simulink model "MARCH_v1_4"  (R2016a)
settings: Solver=FixedStepDiscrete  StartTime=0.0  StopTime=inf  FixedStep=0.001  RelTol=1e-3
PostLoadFcn:
  | build_location = fullfile(fileparts(which(bdroot)),'build');
  | 
  | set_param(0, 'CacheFolder', build_location);
  | set_param(0, 'CodeGenFolder', build_location);
InitFcn:
  | % Change dir to model location
  | cd(fileparts(which(bdroot)));
  | 
  | % Run init script
  | init_model;
  | 
  | load db.mat
  | initialize_model_param
StartFcn:
  | % Make sure we always move back to model folder
  | cd(fileparts(which(bdroot)));
StopFcn:
  | % Make sure we always move back to model folder
  | cd(fileparts(which(bdroot)));
model workspace (MAT data in the model file):
  localValue = 1
  targetValue = 0
libraries: xpcethercatlib x57, slrtlib x7, dspnetwork x1, aerolibanimutils x1
(part 1 of 2)
CloseFcn:
  | % Make sure we always move back to model folder
  | cd(fileparts(which(bdroot)));
  | 
  | set_param(0, 'CacheFolder', '');
  | set_param(0, 'CodeGenFolder', '');
PauseFcn:
  | % Make sure we always move back to model folder
  | cd(fileparts(which(bdroot)));
ContinueFcn:
  | % Make sure we always move back to model folder
  | cd(fileparts(which(bdroot)));
settings Model: Creator=rtheyyun  LastModifiedBy=rafae
settings SolverCC: EnableConcurrentExecution=on  ConcurrentTasks=on
settings DataIOCC: LimitDataPoints=on  SaveFinalState=on  SaveFormat=StructureWithTime  SignalLoggingSaveFormat=ModelDataLogs  InspectSignalLogs=on
settings OptimizationCC: BlockReduction=off  OptimizeBlockIOStorage=off  BufferReuse=off  GlobalBufferReuse=off  ExpressionFolding=off  ExpressionDepthLimit=2147483647  LocalBlockOutputs=off
settings DebuggingCC: ReadBeforeWriteMsg=DisableAll  WriteAfterWriteMsg=DisableAll  WriteAfterReadMsg=DisableAll  UnderspecifiedInitializationDetection=Classic  MergeDetectMultiDrivingBlocksExec=none  SolverPrmCheckMsg=warning  InheritedTsInSrcMsg=none  FcnCallInpInsideContextMsg=UseLocalSettings  AllowSymbolicDim=off  StateNameClashWarn=warning
settings HardwareCC: ProdBitPerPointer=32  ProdLargestAtomicFloat=None  ProdWordSize=32  ProdLongLongMode=on  ProdHWDeviceType=Generic->32-bit x86 compatible
settings ModelReferenceCC: UpdateModelReferenceTargets=Force  PropagateSignalLabelsOutOfModel=off
settings RTWCC: SystemTargetFile=slrt.tlc  TemplateMakefile=slrt_default_tmf  Description=Simulink Real-Time  RTWVerbose=off
settings TargetCC: CodeReplacementLibrary=XPC_BLAS  ParMdlRefBuildCompliant=on  ConcurrentExecutionCompliant=on  MatFileLogging=on  MATLABClassNameForMDSCustomization=xpcAperiodicCustomization
settings ConfigComp: CovModelRefEnable=Off  CovSFcnEnable=off

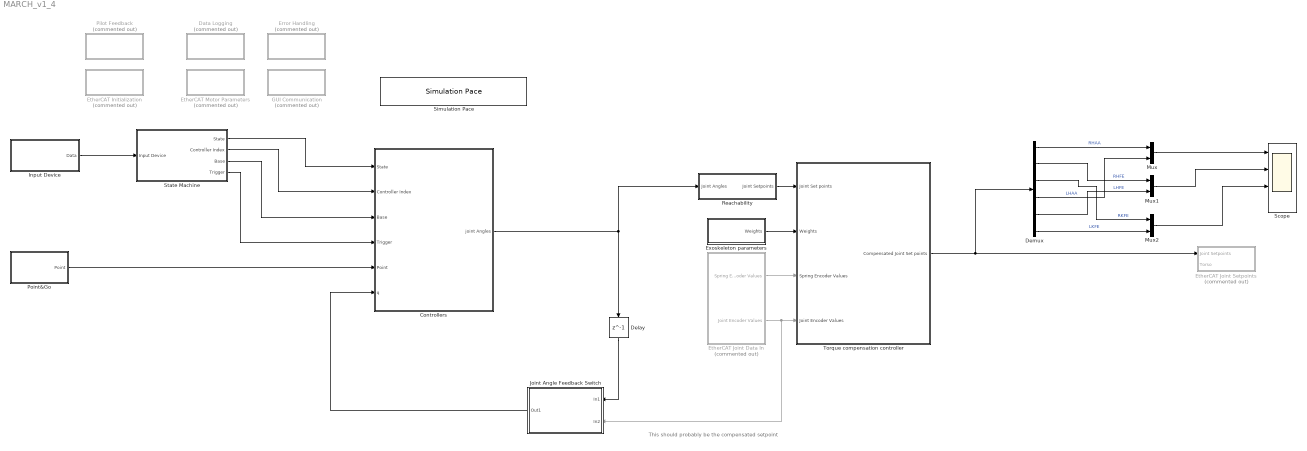
== system MARCH_v1_4 ==
  note: This should probably be the compensated setpoint
  Controllers : Subsystem
  Data Logging : Subsystem  Commented=on
  Delay : Delay  DelayLength=1
  Demux : Demux  Outputs=6
  Error Handling : Subsystem  Commented=on
  EtherCAT Initialization : Subsystem  Commented=on
  EtherCAT Joint Data In : Subsystem  Commented=on
  EtherCAT Joint Setpoints : Subsystem  Commented=on
  EtherCAT Motor Parameters : Subsystem  Commented=on
  Exoskeleton parameters : Subsystem
  GUI Communication : Subsystem  Commented=on
  Input Device : Subsystem
  Joint Angle Feedback Switch : Subsystem
  Mux : Mux  Inputs=2
  Mux1 : Mux  Inputs=2
  Mux2 : Mux  Inputs=2
  Pilot Feedback : Subsystem  Commented=on
  Point&Go : Subsystem
  Reachability : Subsystem
  Scope : Scope  NumInputPorts=4
  Simulation Pace : aerolibanimutils/Simulation Pace  SimulationPace=1  SleepMode=MATLAB Thread  OutputPaceError=off  SampleTime=-1
  State Machine : Subsystem
  Torque compensation controller : Subsystem
  wires:
  Reachability/1(Joint Setpoints) -> Torque compensation controller/1(Joint Set points)
  State Machine/1(State) -> Controllers/1(State)
  EtherCAT Joint Data In/1(Spring Encoder Values) -> Torque compensation controller/3(Spring Encoder Values)
  EtherCAT Joint Data In/2(Joint Encoder Values) -> Joint Angle Feedback Switch/2(In2), Torque compensation controller/4(Joint Encoder Values)
  Exoskeleton parameters/1(Weights) -> Torque compensation controller/2(Weights)
  Controllers/1(joint Angles) -> Reachability/1(Joint Angles), Delay/1
  Joint Angle Feedback Switch/1(Out1) -> Controllers/6(q)
  Delay/1 -> Joint Angle Feedback Switch/1(In1)
  Point&Go/1(Point) -> Controllers/5(Point)
  State Machine/2(Controller Index) -> Controllers/2(Controller Index)
  State Machine/3(Base) -> Controllers/3(Base)
  Input Device/1(Data) -> State Machine/1(Input Device)
  State Machine/4(Trigger) -> Controllers/4(Trigger)
  ? -> Scope/4
  Torque compensation controller/1(Compensated Joint Set points) -> Demux/1, EtherCAT Joint Setpoints/1(Joint Setpoints)
  Demux/1 -> Mux/1  "RHAA"
  Demux/4 -> Mux/2  "LHAA"
  Demux/2 -> Mux1/1  "RHFE"
  Demux/5 -> Mux1/2  "LHFE"
  Demux/3 -> Mux2/1  "RKFE"
  Demux/6 -> Mux2/2  "LKFE"
  Mux/1 -> Scope/1
  Mux1/1 -> Scope/2
  Mux2/1 -> Scope/3

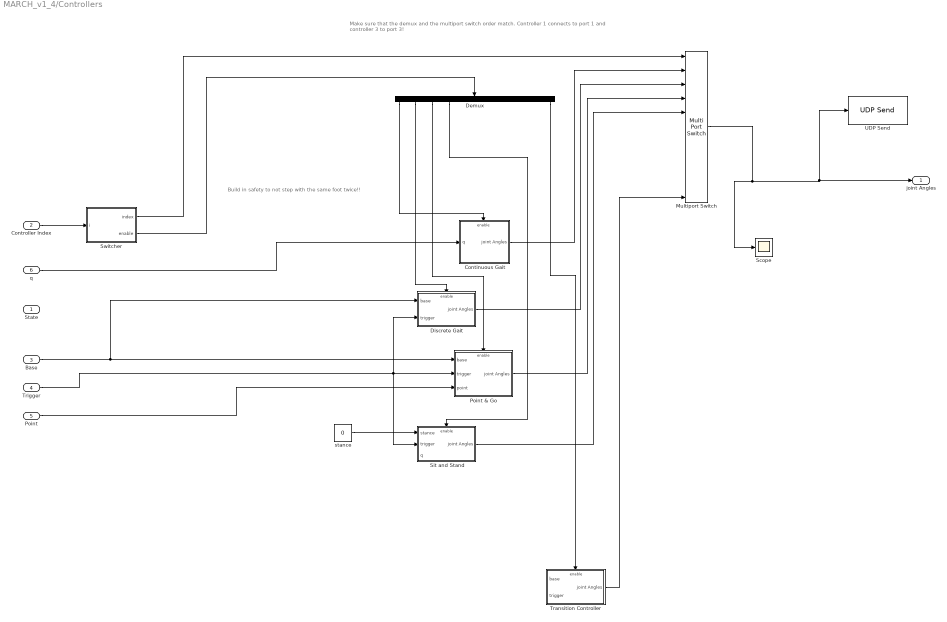
== system MARCH_v1_4/Controllers ==
  note: Build in safety to not step with the same
      | foot twice!!
  note: Make sure that the demux and the multiport switch order match.
      | Controller 1 connects to port 1 and controller 3 to port 3!
  State : Inport
  Controller Index : Inport  Port=2
  Base : Inport  Port=3
  Trigger : Inport  Port=4
  Point : Inport  Port=5
  q : Inport  Port=6
  Continuous Gait : Subsystem
  Demux : Demux  Outputs=10
  Discrete Gait : Subsystem
  Multiport Switch : MultiPortSwitch  Inputs=10
  Point & Go : Subsystem
  Scope : Scope
  Sit and Stand : Subsystem
  Switcher : MATLAB Function  TreatAsAtomicUnit=on
  Transition Controller : Subsystem
  UDP Send : dspnetwork/UDP Send  remoteURL='127.0.0.1'  remotePort=25000  localURL='0.0.0.0'  localPortSource=Automatically determine  localPort=-1  sampletime=-1  separateLengthPort=0
  stance : Constant  Value=0
  joint Angles : Outport
  wires:
  q/1 -> Continuous Gait/1(q)
  Demux/1 -> Continuous Gait/Enable
  Demux/2 -> Discrete Gait/Enable
  Discrete Gait/1(joint Angles) -> Multiport Switch/3
  Controller Index/1 -> Switcher/1(i)
  Switcher/1(index) -> Multiport Switch/1
  Continuous Gait/1(joint Angles) -> Multiport Switch/2
  Multiport Switch/1 -> Scope/1, joint Angles/1, UDP Send/1
  Trigger/1 -> Discrete Gait/2(trigger), Sit and Stand/2(trigger), Point & Go/2(trigger)
  Switcher/2(enable) -> Demux/1
  Base/1 -> Discrete Gait/1(base), Point & Go/1(base)
  Transition Controller/1(joint Angles) -> Multiport Switch/11
  Point & Go/1(joint Angles) -> Multiport Switch/4
  Point/1 -> Point & Go/3(point)
  Demux/3 -> Point & Go/Enable
  Demux/10 -> Transition Controller/Enable
  Demux/4 -> Sit and Stand/Enable
  Sit and Stand/1(joint Angles) -> Multiport Switch/5
  stance/1 -> Sit and Stand/1(stance)

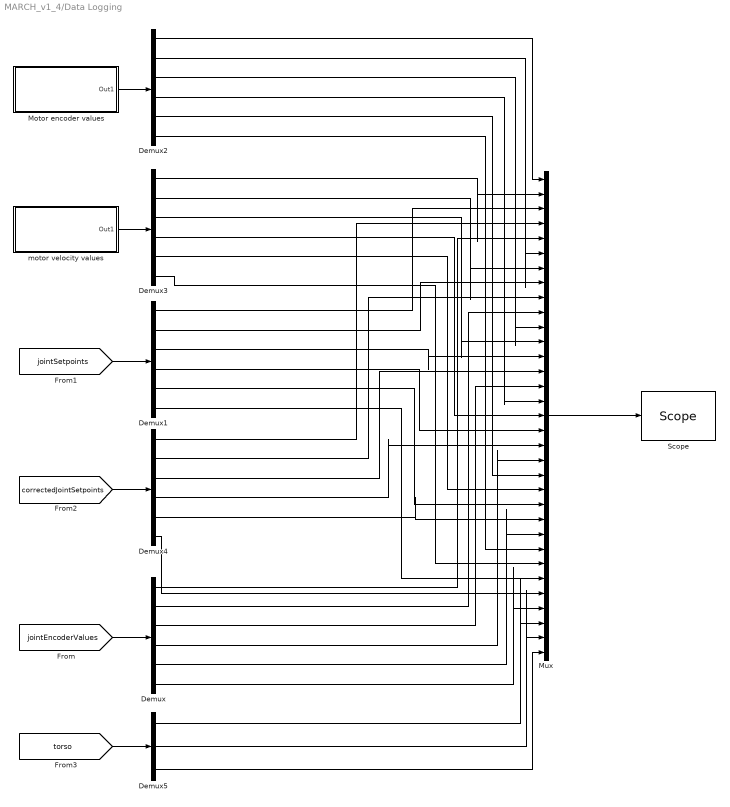
== system MARCH_v1_4/Data Logging ==
  Demux{,1..4} (5 alike) : Demux  Outputs=6
  Demux5 : Demux  Outputs=3
  Motor encoder values : Subsystem
  Mux : Mux  Inputs=33
  "Scope " : slrtlib/Displays and Logging/Scope   scopeno=5  scopetype=File  autostart=on  viewmode=Numerical  formatstr='%15.6f'  grid=on  ylimits=[0,0]  nosamples=250000  noprepostsamples=0  interleave=1  triggermode=FreeRun  triggersignal=1  trigsignalfromport=off  triggerlevel=0.0  triggerslope=Either  triggerscope=1  triggersample=0  filename=datalog.dat  mode=Lazy  writesize=512  autorestart=off  dynamicfilemode=off  maxwritefilesize=512*1024^2
  motor velocity values : Subsystem
  wires:
  Mux/1 -> "Scope "/1
  [jointEncoderValues] -> Demux/1
  [jointSetpoints] -> Demux1/1
  Motor encoder values/1(Out1) -> Demux2/1
  motor velocity values/1(Out1) -> Demux3/1
  Demux2/1 -> Mux/1
  Demux3/1 -> Mux/2
  [correctedJointSetpoints] -> Demux4/1
  [torso] -> Demux5/1
  Demux1/1 -> Mux/3
  Demux4/1 -> Mux/4
  Demux/1 -> Mux/5
  Demux2/2 -> Mux/6
  Demux3/2 -> Mux/7
  Demux1/2 -> Mux/8
  Demux4/2 -> Mux/9
  Demux/2 -> Mux/10
  Demux2/3 -> Mux/11
  Demux3/3 -> Mux/12
  Demux1/3 -> Mux/13
  Demux4/3 -> Mux/14
  Demux/3 -> Mux/15
  Demux2/4 -> Mux/16
  Demux2/6 -> Mux/26
  Demux3/4 -> Mux/17
  Demux1/4 -> Mux/18
  Demux4/4 -> Mux/19
  Demux/4 -> Mux/20
  Demux2/5 -> Mux/21
  Demux3/5 -> Mux/22
  Demux1/5 -> Mux/23
  Demux4/5 -> Mux/24
  Demux/5 -> Mux/25
  Demux3/6 -> Mux/27
  Demux1/6 -> Mux/28
  Demux5/3 -> Mux/33
  Demux5/2 -> Mux/32
  Demux5/1 -> Mux/31
  Demux/6 -> Mux/30
  Demux4/6 -> Mux/29

== system MARCH_v1_4/Error Handling ==

== system MARCH_v1_4/EtherCAT Initialization ==
  "EtherCAT Init " : xpcethercatlib/EtherCAT Init   Priority=0  config_file=D:\Software\MATLAB\simulink-models\EtherCAT Config files\quad_slave_both_legs_v1.0.xml  device_id=0  pci_bus=2  pci_slot=0  dctuning=0  enaDebug=off  enaDC=on  errLink=off  masterDbg=off  stateChgDbg=off  baseClock=off  masterCfg=off  logFile='c:\dbglog.txt'  sample_time=0.001000
  Terminator : Terminator
  wires:
  "EtherCAT Init "/1 -> Terminator/1

== system MARCH_v1_4/EtherCAT Joint Data In ==
  Data Type Conversion : DataTypeConversion  OutDataTypeStr=double
  Joint Encoder EtherCAT : Subsystem  Commented=on
  MATLAB Function : MATLAB Function  TreatAsAtomicUnit=on
  Scope 1 : slrtlib/Displays and Logging/Scope   Commented=on  scopeno=8  scopetype=Target  autostart=on  viewmode=Numerical  formatstr='%15.6f'  grid=on  ylimits=[0,0]  nosamples=3  noprepostsamples=0  interleave=1  triggermode=FreeRun  triggersignal=1  trigsignalfromport=off  triggerlevel=0.0  triggerslope=Either  triggerscope=1  triggersample=0  filename=data.dat  mode=Lazy  writesize=512  autorestart=off  dynamicfilemode=off  maxwritefilesize=512*1024^2
  Scope 2 : slrtlib/Displays and Logging/Scope   Commented=on  scopeno=3  scopetype=Target  autostart=on  viewmode=Numerical  formatstr='%15.6f'  grid=on  ylimits=[0,0]  nosamples=3  noprepostsamples=0  interleave=1  triggermode=FreeRun  triggersignal=1  trigsignalfromport=off  triggerlevel=0.0  triggerslope=Either  triggerscope=1  triggersample=0  filename=data.dat  mode=Lazy  writesize=512  autorestart=off  dynamicfilemode=off  maxwritefilesize=512*1024^2
  Spring Encoder EtherCAT : Subsystem  Commented=on
  Spring Encoder Values : Outport
  Joint Encoder Values : Outport  Port=2
  tag scope: jointEncoderValues=global
  wires:
  Spring Encoder EtherCAT/1(Spring Encoder Values) -> Spring Encoder Values/1
  Joint Encoder EtherCAT/1(Joint Encoder Values) -> Data Type Conversion/1, Scope 2/1, [jointEncoderValues]
  MATLAB Function/1(angles) -> Scope 1/1, Joint Encoder Values/1
  Data Type Conversion/1 -> MATLAB Function/1(encoderValue)

== system MARCH_v1_4/EtherCAT Joint Setpoints ==
  Joint Setpoints : Inport
  Torso : Inport  Port=2
  Subsystem : Subsystem
  exoskeleton : Subsystem
  wires:
  Joint Setpoints/1 -> exoskeleton/1(Joint setpoints), Subsystem/1(Joint Setpoints)
  Torso/1 -> Subsystem/2(Torso)

== system MARCH_v1_4/EtherCAT Motor Parameters ==
  LHFE : Subsystem
  LKFE : Subsystem
  RHFE : Subsystem
  RKFE : Subsystem

== system MARCH_v1_4/Exoskeleton parameters ==
  Constant : Constant
  Weights : Outport
  wires:
  Constant/1 -> Weights/1

== system MARCH_v1_4/GUI Communication ==

== system MARCH_v1_4/Input Device ==
  EtherCAT Input Device : Subsystem  Commented=on
  Left Safety : Constant  Value=0
  Left Trigger : Constant  Value=0
  Local : Constant  Value=localValue
  Mux : Mux  Inputs=6
  Right Safety : Constant  Value=0
  Right Scroll Click : Constant  Value=0
  Right Scroll Position : Constant
  Right Trigger : Constant  Value=0
  Switch : Switch  Criteria=u2 ~= 0
  Data : Outport
  wires:
  Right Scroll Position/1 -> Mux/4
  Mux/1 -> Switch/1
  Right Trigger/1 -> Mux/1
  Switch/1 -> Data/1
  Right Safety/1 -> Mux/2
  Right Scroll Click/1 -> Mux/3
  Left Trigger/1 -> Mux/5
  Local/1 -> Switch/2
  Left Safety/1 -> Mux/6
  EtherCAT Input Device/1(Input Device) -> Switch/3

== system MARCH_v1_4/Joint Angle Feedback Switch ==
  In1 : Inport
  In2 : Inport  Port=2
  Local : Constant  Value=localValue
  Switch : Switch  Criteria=u2 ~= 0
  Out1 : Outport
  wires:
  In2/1 -> Switch/3
  Switch/1 -> Out1/1
  In1/1 -> Switch/1
  Local/1 -> Switch/2

== system MARCH_v1_4/Pilot Feedback ==

== system MARCH_v1_4/Point&Go ==
  EtherCAT Point&Go : Subsystem  Commented=on
  Local : Constant  Value=localValue
  Point & Go Point : Constant  Value=[0.7 -0.3]
  Switch : Switch  Criteria=u2 ~= 0
  Point : Outport
  wires:
  EtherCAT Point&Go/1(Point&Go Data) -> Switch/3
  Local/1 -> Switch/2
  Switch/1 -> Point/1
  Point & Go Point/1 -> Switch/1

== system MARCH_v1_4/Reachability ==
  Joint Angles : Inport
  Data Type Conversion : DataTypeConversion  OutDataTypeStr=uint32
  MATLAB Function : MATLAB Function  Commented=on  TreatAsAtomicUnit=on
  Terminator2 : Terminator
  Joint Setpoints : Outport
  tag scope: jointSetpoints=global
  wires:
  MATLAB Function/2(err) -> Terminator2/1
  Data Type Conversion/1 -> [jointSetpoints]
  Joint Angles/1 -> Data Type Conversion/1, Joint Setpoints/1

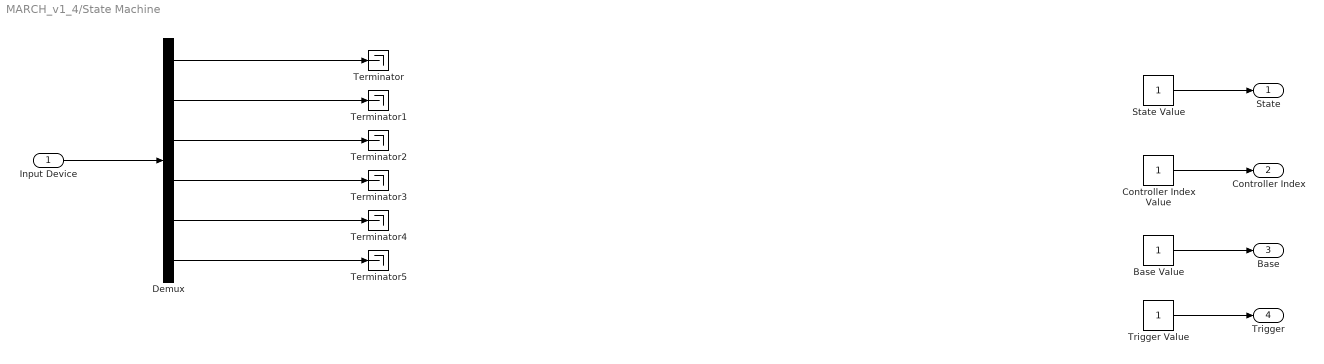
== system MARCH_v1_4/State Machine ==
  Input Device : Inport
  Base Value : Constant
  Controller Index Value : Constant
  Demux : Demux  Outputs=6
  State Value : Constant
  Terminator{,1..5} (6 alike) : Terminator
  Trigger Value : Constant
  State : Outport
  Controller Index : Outport  Port=2
  Base : Outport  Port=3
  Trigger : Outport  Port=4
  wires:
  State Value/1 -> State/1
  Input Device/1 -> Demux/1
  Controller Index Value/1 -> Controller Index/1
  Base Value/1 -> Base/1
  Trigger Value/1 -> Trigger/1
  Demux/1 -> Terminator/1
  Demux/2 -> Terminator1/1
  Demux/3 -> Terminator2/1
  Demux/4 -> Terminator3/1
  Demux/5 -> Terminator4/1
  Demux/6 -> Terminator5/1

== system MARCH_v1_4/Torque compensation controller ==
  Joint Set points : Inport
  Weights : Inport  Port=2
  Spring Encoder Values : Inport  Port=3
  Joint Encoder Values : Inport  Port=4
  Terminator : Terminator
  Terminator1 : Terminator
  Terminator2 : Terminator
  Compensated Joint Set points : Outport
  wires:
  Joint Set points/1 -> Compensated Joint Set points/1
  Joint Encoder Values/1 -> Terminator2/1
  Spring Encoder Values/1 -> Terminator1/1
  Weights/1 -> Terminator/1

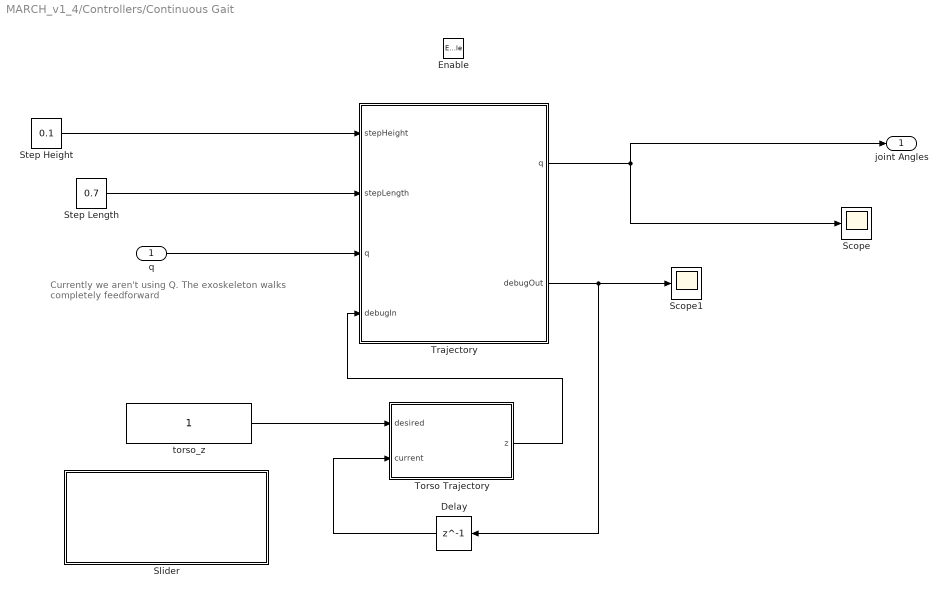
== system MARCH_v1_4/Controllers/Continuous Gait ==
  note: Currently we aren't using Q. The exoskeleton walks completely feedforward
  q : Inport
  Enable : EnablePort
  Delay : Delay  DelayLength=1  InitialCondition=1
  Scope : Scope
  Scope1 : Scope
  Slider : Subsystem  DialogController=hmiCreateDDGDialog  IsWebBlock=on  mask(MWDashboardBlock){webBlockId=08960381-2fc9-439b-949a-5d55ec4678c5, webBlockType=slider, ShowInLibBrowser=on, ShowInitialText=on, HMISrcModelName=MARCH_v1_4}
      mask prompts: webBlockId "WebBlock Id"; webBlockType "WebBlock Type"; HMISrcModelName "Source Model"
      mask Help: helpview([docroot '/mapfiles/simulink.map'], 'hmi_slider')
      mask Display:
      | if strcmp(get_param(bdroot(gcb),'BlockDiagramType'), 'library')
      |     image([(matlabroot) '/toolbox/simulink/hmi/icons/Slider.png']);
      | end
  Step Height : Constant  Value=0.1
  Step Length : Constant  Value=0.7
  Torso Trajectory : MATLAB Function  TreatAsAtomicUnit=on
  Trajectory : MATLAB Function  TreatAsAtomicUnit=on
  torso_z : Constant
  joint Angles : Outport
  wires:
  Step Length/1 -> Trajectory/2(stepLength)
  Trajectory/1(q) -> joint Angles/1, Scope/1
  q/1 -> Trajectory/3("q ")
  Step Height/1 -> Trajectory/1(stepHeight)
  Trajectory/2(debugOut) -> Delay/1, Scope1/1
  torso_z/1 -> Torso Trajectory/1(desired)
  Torso Trajectory/1(z) -> Trajectory/4(debugIn)
  Delay/1 -> Torso Trajectory/2(current)

== system MARCH_v1_4/Controllers/Discrete Gait ==
  base : Inport
  trigger : Inport  Port=2
  Enable : EnablePort
  Delay : Delay  DelayLength=1  InitialCondition=1
  Scope : Scope
  Scope1 : Scope
  Slider : Subsystem  DialogController=hmiCreateDDGDialog  IsWebBlock=on  mask(MWDashboardBlock){webBlockId=bfbe03fb-e7b8-42bf-a623-efab1dfdd155, webBlockType=slider, ShowInLibBrowser=on, ShowInitialText=on, HMISrcModelName=MARCH_v1_4}
      mask prompts: webBlockId "WebBlock Id"; webBlockType "WebBlock Type"; HMISrcModelName "Source Model"
      mask Help: helpview([docroot '/mapfiles/simulink.map'], 'hmi_slider')
      mask Display:
      | if strcmp(get_param(bdroot(gcb),'BlockDiagramType'), 'library')
      |     image([(matlabroot) '/toolbox/simulink/hmi/icons/Slider.png']);
      | end
  Torso Trajectory : MATLAB Function  TreatAsAtomicUnit=on
  Trajectory : MATLAB Function  TreatAsAtomicUnit=on
  torso_z : Constant
  joint Angles : Outport
  wires:
  Trajectory/1(q) -> joint Angles/1, Scope/1
  trigger/1 -> Trajectory/2(trigger)
  Trajectory/2(debugOut) -> Delay/1, Scope1/1
  torso_z/1 -> Torso Trajectory/1(desired)
  Torso Trajectory/1(z) -> Trajectory/4(debugIn)
  Delay/1 -> Torso Trajectory/2(current)
  base/1 -> Trajectory/1(base)

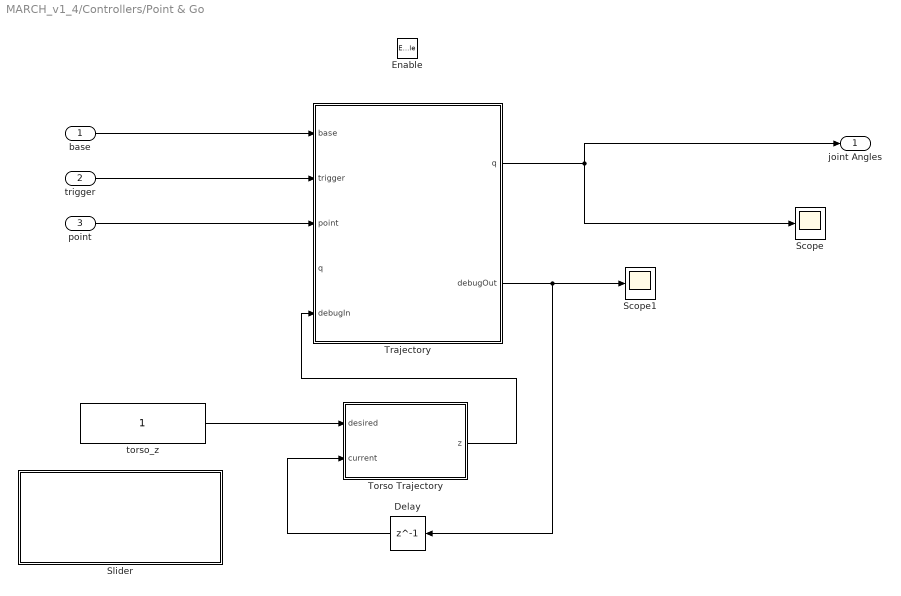
== system MARCH_v1_4/Controllers/Point & Go ==
  base : Inport
  trigger : Inport  Port=2
  point : Inport  Port=3
  Enable : EnablePort
  Delay : Delay  DelayLength=1  InitialCondition=1
  Scope : Scope
  Scope1 : Scope
  Slider : Subsystem  DialogController=hmiCreateDDGDialog  IsWebBlock=on  mask(MWDashboardBlock){webBlockId=86d33f0a-5aea-492b-afd2-e04e6c4ab60f, webBlockType=slider, ShowInLibBrowser=on, ShowInitialText=on, HMISrcModelName=MARCH_v1_4}
      mask prompts: webBlockId "WebBlock Id"; webBlockType "WebBlock Type"; HMISrcModelName "Source Model"
      mask Help: helpview([docroot '/mapfiles/simulink.map'], 'hmi_slider')
      mask Display:
      | if strcmp(get_param(bdroot(gcb),'BlockDiagramType'), 'library')
      |     image([(matlabroot) '/toolbox/simulink/hmi/icons/Slider.png']);
      | end
  Torso Trajectory : MATLAB Function  TreatAsAtomicUnit=on
  Trajectory : MATLAB Function  TreatAsAtomicUnit=on
  torso_z : Constant
  joint Angles : Outport
  wires:
  Trajectory/1(q) -> joint Angles/1, Scope/1
  trigger/1 -> Trajectory/2(trigger)
  Trajectory/2(debugOut) -> Delay/1, Scope1/1
  torso_z/1 -> Torso Trajectory/1(desired)
  Torso Trajectory/1(z) -> Trajectory/5(debugIn)
  Delay/1 -> Torso Trajectory/2(current)
  base/1 -> Trajectory/1(base)
  point/1 -> Trajectory/3(point)

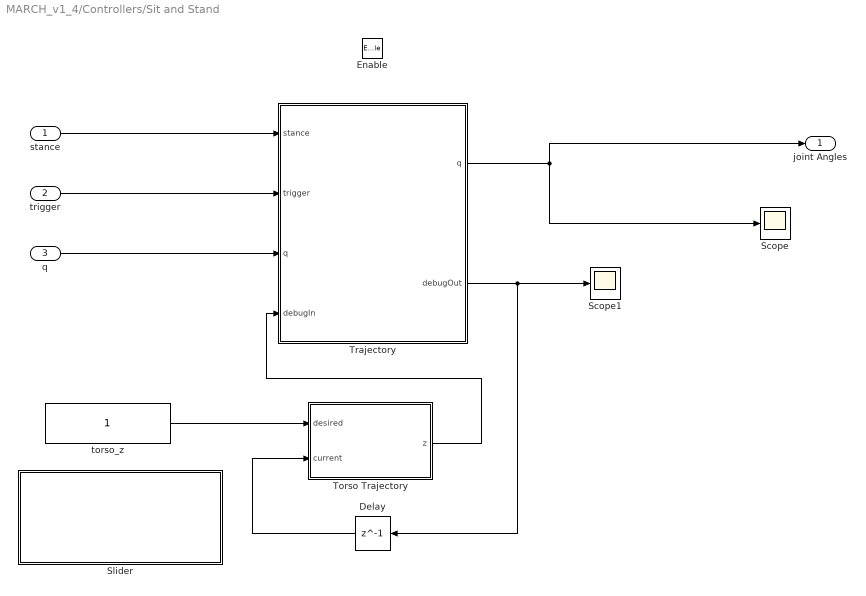
== system MARCH_v1_4/Controllers/Sit and Stand ==
  stance : Inport
  trigger : Inport  Port=2
  "q " : Inport  Port=3
  Enable : EnablePort
  Delay : Delay  DelayLength=1  InitialCondition=1
  Scope : Scope
  Scope1 : Scope
  Slider : Subsystem  DialogController=hmiCreateDDGDialog  IsWebBlock=on  mask(MWDashboardBlock){webBlockId=b1d2559e-7f74-4a22-bcb5-6ee8e71e9ba8, webBlockType=slider, ShowInLibBrowser=on, ShowInitialText=on, HMISrcModelName=MARCH_v1_4}
      mask prompts: webBlockId "WebBlock Id"; webBlockType "WebBlock Type"; HMISrcModelName "Source Model"
      mask Help: helpview([docroot '/mapfiles/simulink.map'], 'hmi_slider')
      mask Display:
      | if strcmp(get_param(bdroot(gcb),'BlockDiagramType'), 'library')
      |     image([(matlabroot) '/toolbox/simulink/hmi/icons/Slider.png']);
      | end
  Torso Trajectory : MATLAB Function  TreatAsAtomicUnit=on
  Trajectory : MATLAB Function  TreatAsAtomicUnit=on
  torso_z : Constant
  joint Angles : Outport
  wires:
  Trajectory/1(q) -> joint Angles/1, Scope/1
  trigger/1 -> Trajectory/2(trigger)
  Trajectory/2(debugOut) -> Delay/1, Scope1/1
  torso_z/1 -> Torso Trajectory/1(desired)
  Torso Trajectory/1(z) -> Trajectory/4(debugIn)
  Delay/1 -> Torso Trajectory/2(current)
  stance/1 -> Trajectory/1(stance)
  "q "/1 -> Trajectory/3("q ")

== system MARCH_v1_4/Controllers/Transition Controller ==
  base : Inport
  trigger : Inport  Port=2
  Enable : EnablePort
  Delay : Delay  DelayLength=1  InitialCondition=1
  Scope : Scope
  Scope1 : Scope
  Slider : Subsystem  DialogController=hmiCreateDDGDialog  IsWebBlock=on  mask(MWDashboardBlock){webBlockId=004e6a24-cc7d-4bcf-a064-e862a4729289, webBlockType=slider, ShowInLibBrowser=on, ShowInitialText=on, HMISrcModelName=MARCH_v1_4}
      mask prompts: webBlockId "WebBlock Id"; webBlockType "WebBlock Type"; HMISrcModelName "Source Model"
      mask Help: helpview([docroot '/mapfiles/simulink.map'], 'hmi_slider')
      mask Display:
      | if strcmp(get_param(bdroot(gcb),'BlockDiagramType'), 'library')
      |     image([(matlabroot) '/toolbox/simulink/hmi/icons/Slider.png']);
      | end
  Torso Trajectory : MATLAB Function  TreatAsAtomicUnit=on
  Trajectory : MATLAB Function  TreatAsAtomicUnit=on
  torso_z : Constant
  joint Angles : Outport
  wires:
  Trajectory/1(q) -> joint Angles/1, Scope/1
  trigger/1 -> Trajectory/2(trigger)
  Trajectory/2(debugOut) -> Delay/1, Scope1/1
  torso_z/1 -> Torso Trajectory/1(desired)
  Torso Trajectory/1(z) -> Trajectory/4(debugIn)
  Delay/1 -> Torso Trajectory/2(current)
  base/1 -> Trajectory/1(base)

== system MARCH_v1_4/Data Logging/Motor encoder values ==
  Data Type Conversion : DataTypeConversion  OutDataTypeStr=uint32
  EtherCAT PDO Receive1 : xpcethercatlib/EtherCAT PDO Receive  Priority=2  sig_name=RHFE.Inputs.motorAngle  sig_offset=12528  sig_type=uint16  type_size=16  sig_dim=1  device_id=0  sample_time=0.001000
  EtherCAT PDO Receive2 : xpcethercatlib/EtherCAT PDO Receive  Priority=2  sig_name=RHFE.Inputs.motorAngle  sig_offset=12528  sig_type=uint16  type_size=16  sig_dim=1  device_id=0  sample_time=0.001000
  EtherCAT PDO Receive3 : xpcethercatlib/EtherCAT PDO Receive  Priority=2  sig_name=LHFE.Inputs.motorAngle  sig_offset=240  sig_type=uint16  type_size=16  sig_dim=1  device_id=0  sample_time=0.001000
  EtherCAT PDO Receive4 : xpcethercatlib/EtherCAT PDO Receive  Priority=2  sig_name=LHFE.Inputs.motorAngle  sig_offset=240  sig_type=uint16  type_size=16  sig_dim=1  device_id=0  sample_time=0.001000
  EtherCAT PDO Receive5 : xpcethercatlib/EtherCAT PDO Receive  Priority=2  sig_name=RKFE.Inputs.motorAngle  sig_offset=12816  sig_type=uint16  type_size=16  sig_dim=1  device_id=0  sample_time=0.001000
  EtherCAT PDO Receive7 : xpcethercatlib/EtherCAT PDO Receive  Priority=2  sig_name=LKFE.Inputs.motorAngle  sig_offset=528  sig_type=uint16  type_size=16  sig_dim=1  device_id=0  sample_time=0.001000
  Mux1 : Mux  Inputs=6
  Out1 : Outport
  wires:
  EtherCAT PDO Receive4/1 -> Mux1/4
  EtherCAT PDO Receive5/1 -> Mux1/3
  EtherCAT PDO Receive7/1 -> Mux1/6
  Mux1/1 -> Data Type Conversion/1
  EtherCAT PDO Receive1/1 -> Mux1/1
  EtherCAT PDO Receive3/1 -> Mux1/5
  EtherCAT PDO Receive2/1 -> Mux1/2
  Data Type Conversion/1 -> Out1/1

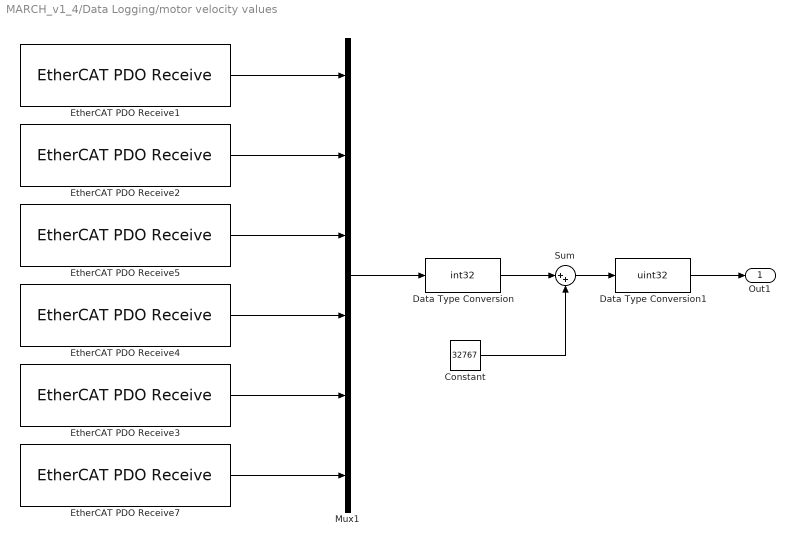
== system MARCH_v1_4/Data Logging/motor velocity values ==
  Constant : Constant  Value=32767
  Data Type Conversion : DataTypeConversion  OutDataTypeStr=int32
  Data Type Conversion1 : DataTypeConversion  OutDataTypeStr=uint32
  EtherCAT PDO Receive1 : xpcethercatlib/EtherCAT PDO Receive  Priority=2  sig_name=RHFE.Inputs.motorVelocity  sig_offset=12544  sig_type=int16  type_size=16  sig_dim=1  device_id=0  sample_time=0.001000
  EtherCAT PDO Receive2 : xpcethercatlib/EtherCAT PDO Receive  Priority=2  sig_name=RHFE.Inputs.motorVelocity  sig_offset=12544  sig_type=int16  type_size=16  sig_dim=1  device_id=0  sample_time=0.001000
  EtherCAT PDO Receive3 : xpcethercatlib/EtherCAT PDO Receive  Priority=2  sig_name=LHFE.Inputs.motorVelocity  sig_offset=256  sig_type=int16  type_size=16  sig_dim=1  device_id=0  sample_time=0.001000
  EtherCAT PDO Receive4 : xpcethercatlib/EtherCAT PDO Receive  Priority=2  sig_name=LHFE.Inputs.motorVelocity  sig_offset=256  sig_type=int16  type_size=16  sig_dim=1  device_id=0  sample_time=0.001000
  EtherCAT PDO Receive5 : xpcethercatlib/EtherCAT PDO Receive  Priority=2  sig_name=RKFE.Inputs.motorVelocity  sig_offset=12832  sig_type=int16  type_size=16  sig_dim=1  device_id=0  sample_time=0.001000
  EtherCAT PDO Receive7 : xpcethercatlib/EtherCAT PDO Receive  Priority=2  sig_name=LKFE.Inputs.motorVelocity  sig_offset=544  sig_type=int16  type_size=16  sig_dim=1  device_id=0  sample_time=0.001000
  Mux1 : Mux  Inputs=6
  Sum : Sum  Inputs=|++
  Out1 : Outport
  wires:
  EtherCAT PDO Receive2/1 -> Mux1/2
  EtherCAT PDO Receive3/1 -> Mux1/5
  EtherCAT PDO Receive1/1 -> Mux1/1
  Mux1/1 -> Data Type Conversion/1
  EtherCAT PDO Receive7/1 -> Mux1/6
  EtherCAT PDO Receive5/1 -> Mux1/3
  EtherCAT PDO Receive4/1 -> Mux1/4
  Constant/1 -> Sum/2
  Data Type Conversion/1 -> Sum/1
  Sum/1 -> Data Type Conversion1/1
  Data Type Conversion1/1 -> Out1/1

== system MARCH_v1_4/EtherCAT Joint Data In/Joint Encoder EtherCAT ==
  EtherCAT PDO Receive10 : xpcethercatlib/EtherCAT PDO Receive  Priority=2  sig_name=LHFE.Inputs.jointAngle  sig_offset=208  sig_type=uint32  type_size=32  sig_dim=1  device_id=0  sample_time=0.001000
  EtherCAT PDO Receive11 : xpcethercatlib/EtherCAT PDO Receive  Priority=2  sig_name=LKFE.Inputs.jointAngle  sig_offset=496  sig_type=uint32  type_size=32  sig_dim=1  device_id=0  sample_time=0.001000
  EtherCAT PDO Receive6 : xpcethercatlib/EtherCAT PDO Receive  Priority=2  Commented=on  sig_name=LHFE.Inputs.jointAngle  sig_offset=208  sig_type=uint32  type_size=32  sig_dim=1  device_id=0  sample_time=0.001000
  EtherCAT PDO Receive7 : xpcethercatlib/EtherCAT PDO Receive  Priority=2  sig_name=RHFE.Inputs.jointAngle  sig_offset=12496  sig_type=uint32  type_size=32  sig_dim=1  device_id=0  sample_time=0.001000
  EtherCAT PDO Receive8 : xpcethercatlib/EtherCAT PDO Receive  Priority=2  sig_name=RKFE.Inputs.jointAngle  sig_offset=12784  sig_type=uint32  type_size=32  sig_dim=1  device_id=0  sample_time=0.001000
  EtherCAT PDO Receive9 : xpcethercatlib/EtherCAT PDO Receive  Priority=2  Commented=on  sig_name=LHFE.Inputs.jointAngle  sig_offset=208  sig_type=uint32  type_size=32  sig_dim=1  device_id=0  sample_time=0.001000
  Mux1 : Mux  Inputs=6
  Joint Encoder Values : Outport
  wires:
  EtherCAT PDO Receive8/1 -> Mux1/3
  EtherCAT PDO Receive9/1 -> Mux1/4
  EtherCAT PDO Receive7/1 -> Mux1/2
  EtherCAT PDO Receive6/1 -> Mux1/1
  EtherCAT PDO Receive10/1 -> Mux1/5
  EtherCAT PDO Receive11/1 -> Mux1/6
  Mux1/1 -> Joint Encoder Values/1

== system MARCH_v1_4/EtherCAT Joint Data In/Spring Encoder EtherCAT ==
  EtherCAT PDO Receive{,1..5} (6 alike) : xpcethercatlib/EtherCAT PDO Receive  Priority=2  sig_name=LHFE.Inputs.jointAngle  sig_offset=208  sig_type=uint32  type_size=32  sig_dim=1  device_id=0  sample_time=0.001000
  Mux : Mux  Inputs=6
  Spring Encoder Values : Outport
  wires:
  EtherCAT PDO Receive2/1 -> Mux/3
  EtherCAT PDO Receive4/1 -> Mux/5
  Mux/1 -> Spring Encoder Values/1
  EtherCAT PDO Receive5/1 -> Mux/6
  EtherCAT PDO Receive1/1 -> Mux/2
  EtherCAT PDO Receive/1 -> Mux/1
  EtherCAT PDO Receive3/1 -> Mux/4

== system MARCH_v1_4/EtherCAT Joint Setpoints/Subsystem ==
  Joint Setpoints : Inport
  Torso : Inport  Port=2
  Data Type Conversion : DataTypeConversion  OutDataTypeStr=uint32
  Data Type Conversion1 : DataTypeConversion  OutDataTypeStr=uint32
  tag scope: correctedJointSetpoints=global, torso=global
  wires:
  Joint Setpoints/1 -> Data Type Conversion/1
  Torso/1 -> Data Type Conversion1/1
  Data Type Conversion/1 -> [correctedJointSetpoints]
  Data Type Conversion1/1 -> [torso]

== system MARCH_v1_4/EtherCAT Joint Setpoints/exoskeleton ==
  Joint setpoints : Inport
  Data Type Conversion : DataTypeConversion  OutDataTypeStr=uint32
  EtherCAT Joint Communication : Subsystem  Commented=on
  MATLAB Function : MATLAB Function  Commented=on  TreatAsAtomicUnit=on
  "Scope " : slrtlib/Displays and Logging/Scope   Commented=on  scopeno=2  scopetype=Target  autostart=on  viewmode=Numerical  formatstr='%15.6f'  grid=on  ylimits=[0,0]  nosamples=3  noprepostsamples=0  interleave=1  triggermode=FreeRun  triggersignal=1  trigsignalfromport=off  triggerlevel=0.0  triggerslope=Either  triggerscope=1  triggersample=0  filename=data.dat  mode=Lazy  writesize=512  autorestart=off  dynamicfilemode=off  maxwritefilesize=512*1024^2
  Scope 1 : slrtlib/Displays and Logging/Scope   Commented=on  scopeno=1  scopetype=Target  autostart=on  viewmode=Graphical sliding  formatstr='%15.6f'  grid=on  ylimits=[0,0]  nosamples=25000  noprepostsamples=0  interleave=1  triggermode=FreeRun  triggersignal=1  trigsignalfromport=off  triggerlevel=0.0  triggerslope=Either  triggerscope=1  triggersample=0  filename=data.dat  mode=Lazy  writesize=512  autorestart=off  dynamicfilemode=off  maxwritefilesize=512*1024^2
  Scope 2 : slrtlib/Displays and Logging/Scope   Commented=on  scopeno=6  scopetype=Target  autostart=on  viewmode=Numerical  formatstr='%15.6f'  grid=on  ylimits=[0,0]  nosamples=3  noprepostsamples=0  interleave=1  triggermode=FreeRun  triggersignal=1  trigsignalfromport=off  triggerlevel=0.0  triggerslope=Either  triggerscope=1  triggersample=0  filename=data.dat  mode=Lazy  writesize=512  autorestart=off  dynamicfilemode=off  maxwritefilesize=512*1024^2
  Scope 3 : slrtlib/Displays and Logging/Scope   Commented=on  scopeno=7  scopetype=Target  autostart=on  viewmode=Graphical sliding  formatstr='%15.6f'  grid=on  ylimits=[0,0]  nosamples=25000  noprepostsamples=0  interleave=1  triggermode=FreeRun  triggersignal=1  trigsignalfromport=off  triggerlevel=0.0  triggerslope=Either  triggerscope=1  triggersample=0  filename=data.dat  mode=Lazy  writesize=512  autorestart=off  dynamicfilemode=off  maxwritefilesize=512*1024^2
  wires:
  Data Type Conversion/1 -> EtherCAT Joint Communication/1(Joint Setpoints)
  Joint setpoints/1 -> Scope 1/1, "Scope "/1, Data Type Conversion/1, Scope 3/1, Scope 2/1

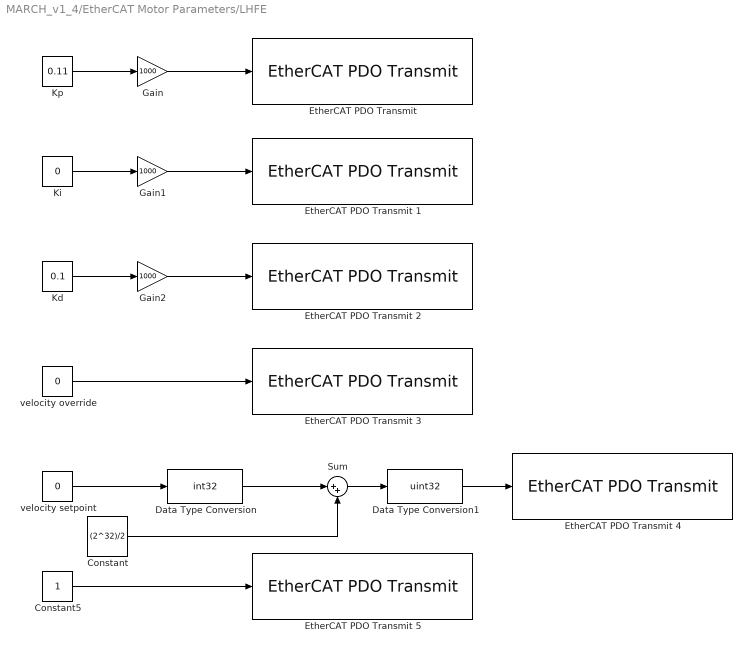
== system MARCH_v1_4/EtherCAT Motor Parameters/LHFE ==
  Constant : Constant  Value=(2^32)/2  VectorParams1D=off  SampleTime=-1
  Constant5 : Constant  OutDataTypeStr=uint32
  Data Type Conversion : DataTypeConversion  OutDataTypeStr=int32
  Data Type Conversion1 : DataTypeConversion  OutDataTypeStr=uint32
  "EtherCAT PDO Transmit " : xpcethercatlib/EtherCAT PDO Transmit   Priority=3  sig_name=LHFE.Outputs.data1  sig_offset=272  sig_type=uint32  type_size=32  sig_dim=1  device_id=0  sample_time=0.001000
  EtherCAT PDO Transmit 1 : xpcethercatlib/EtherCAT PDO Transmit   Priority=3  sig_name=LHFE.Outputs.data2  sig_offset=304  sig_type=uint32  type_size=32  sig_dim=1  device_id=0  sample_time=0.001000
  EtherCAT PDO Transmit 2 : xpcethercatlib/EtherCAT PDO Transmit   Priority=3  sig_name=LHFE.Outputs.data3  sig_offset=336  sig_type=uint32  type_size=32  sig_dim=1  device_id=0  sample_time=0.001000
  EtherCAT PDO Transmit 3 : xpcethercatlib/EtherCAT PDO Transmit   Priority=3  sig_name=LHFE.Outputs.data4  sig_offset=368  sig_type=uint32  type_size=32  sig_dim=1  device_id=0  sample_time=0.001000
  EtherCAT PDO Transmit 4 : xpcethercatlib/EtherCAT PDO Transmit   Priority=3  sig_name=LHFE.Outputs.data0  sig_offset=240  sig_type=uint32  type_size=32  sig_dim=1  device_id=0  sample_time=0.001000
  EtherCAT PDO Transmit 5 : xpcethercatlib/EtherCAT PDO Transmit   Priority=3  sig_name=LHFE.Outputs.data7  sig_offset=464  sig_type=uint32  type_size=32  sig_dim=1  device_id=0  sample_time=0.001000
  Gain : Gain  Gain=1000  OutDataTypeStr=uint32
  Gain1 : Gain  Gain=1000  OutDataTypeStr=uint32
  Gain2 : Gain  Gain=1000  OutDataTypeStr=uint32
  Kd : Constant  Value=0.1  OutDataTypeStr=double
  Ki : Constant  Value=0  OutDataTypeStr=double
  Kp : Constant  Value=0.11  OutDataTypeStr=double
  Sum : Sum  Inputs=|++
  velocity override : Constant  Value=0  OutDataTypeStr=uint32
  velocity setpoint : Constant  Value=0  OutDataTypeStr=int16
  wires:
  Kd/1 -> Gain2/1
  velocity setpoint/1 -> Data Type Conversion/1
  Kp/1 -> Gain/1
  Constant5/1 -> EtherCAT PDO Transmit 5/1
  Ki/1 -> Gain1/1
  velocity override/1 -> EtherCAT PDO Transmit 3/1
  Constant/1 -> Sum/2
  Data Type Conversion/1 -> Sum/1
  Sum/1 -> Data Type Conversion1/1
  Data Type Conversion1/1 -> EtherCAT PDO Transmit 4/1
  Gain/1 -> "EtherCAT PDO Transmit "/1
  Gain1/1 -> EtherCAT PDO Transmit 1/1
  Gain2/1 -> EtherCAT PDO Transmit 2/1

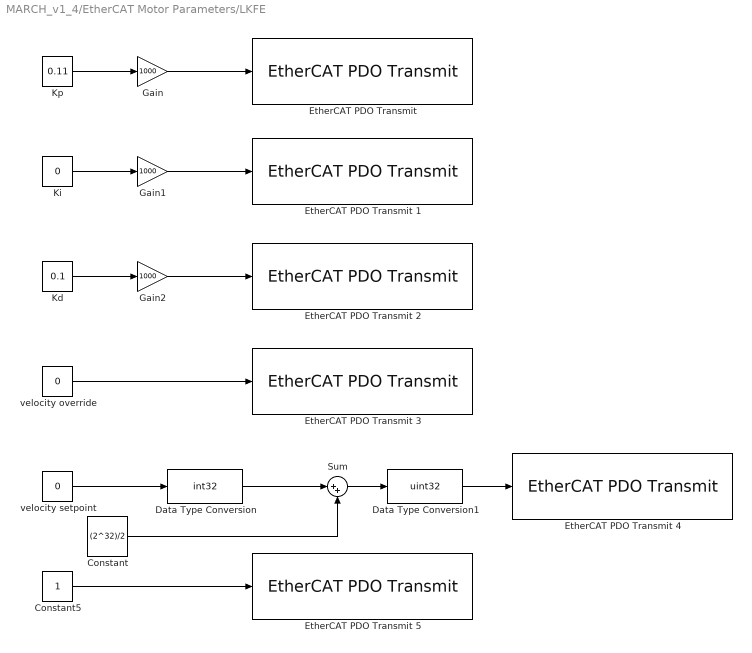
== system MARCH_v1_4/EtherCAT Motor Parameters/LKFE ==
  Constant : Constant  Value=(2^32)/2  VectorParams1D=off  SampleTime=-1
  Constant5 : Constant  OutDataTypeStr=uint32
  Data Type Conversion : DataTypeConversion  OutDataTypeStr=int32
  Data Type Conversion1 : DataTypeConversion  OutDataTypeStr=uint32
  "EtherCAT PDO Transmit " : xpcethercatlib/EtherCAT PDO Transmit   Priority=3  sig_name=LKFE.Outputs.data1  sig_offset=560  sig_type=uint32  type_size=32  sig_dim=1  device_id=0  sample_time=0.001000
  EtherCAT PDO Transmit 1 : xpcethercatlib/EtherCAT PDO Transmit   Priority=3  sig_name=LKFE.Outputs.data2  sig_offset=592  sig_type=uint32  type_size=32  sig_dim=1  device_id=0  sample_time=0.001000
  EtherCAT PDO Transmit 2 : xpcethercatlib/EtherCAT PDO Transmit   Priority=3  sig_name=LKFE.Outputs.data3  sig_offset=624  sig_type=uint32  type_size=32  sig_dim=1  device_id=0  sample_time=0.001000
  EtherCAT PDO Transmit 3 : xpcethercatlib/EtherCAT PDO Transmit   Priority=3  sig_name=LKFE.Outputs.data4  sig_offset=656  sig_type=uint32  type_size=32  sig_dim=1  device_id=0  sample_time=0.001000
  EtherCAT PDO Transmit 4 : xpcethercatlib/EtherCAT PDO Transmit   Priority=3  sig_name=LKFE.Outputs.data0  sig_offset=528  sig_type=uint32  type_size=32  sig_dim=1  device_id=0  sample_time=0.001000
  EtherCAT PDO Transmit 5 : xpcethercatlib/EtherCAT PDO Transmit   Priority=3  sig_name=LKFE.Outputs.data7  sig_offset=752  sig_type=uint32  type_size=32  sig_dim=1  device_id=0  sample_time=0.001000
  Gain : Gain  Gain=1000  OutDataTypeStr=uint32
  Gain1 : Gain  Gain=1000  OutDataTypeStr=uint32
  Gain2 : Gain  Gain=1000  OutDataTypeStr=uint32
  Kd : Constant  Value=0.1  OutDataTypeStr=double
  Ki : Constant  Value=0  OutDataTypeStr=double
  Kp : Constant  Value=0.11  OutDataTypeStr=double
  Sum : Sum  Inputs=|++
  velocity override : Constant  Value=0  OutDataTypeStr=uint32
  velocity setpoint : Constant  Value=0  OutDataTypeStr=int16
  wires:
  Kd/1 -> Gain2/1
  velocity setpoint/1 -> Data Type Conversion/1
  Kp/1 -> Gain/1
  Constant5/1 -> EtherCAT PDO Transmit 5/1
  Ki/1 -> Gain1/1
  velocity override/1 -> EtherCAT PDO Transmit 3/1
  Constant/1 -> Sum/2
  Data Type Conversion/1 -> Sum/1
  Sum/1 -> Data Type Conversion1/1
  Data Type Conversion1/1 -> EtherCAT PDO Transmit 4/1
  Gain/1 -> "EtherCAT PDO Transmit "/1
  Gain1/1 -> EtherCAT PDO Transmit 1/1
  Gain2/1 -> EtherCAT PDO Transmit 2/1

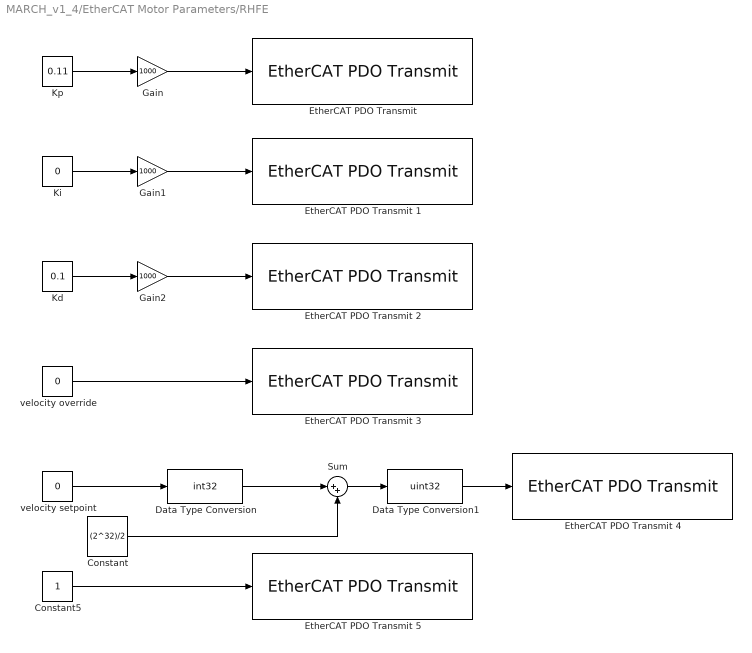
== system MARCH_v1_4/EtherCAT Motor Parameters/RHFE ==
  Constant : Constant  Value=(2^32)/2  VectorParams1D=off  SampleTime=-1
  Constant5 : Constant  OutDataTypeStr=uint32
  Data Type Conversion : DataTypeConversion  OutDataTypeStr=int32
  Data Type Conversion1 : DataTypeConversion  OutDataTypeStr=uint32
  "EtherCAT PDO Transmit " : xpcethercatlib/EtherCAT PDO Transmit   Priority=3  sig_name=RHFE.Outputs.data1  sig_offset=12560  sig_type=uint32  type_size=32  sig_dim=1  device_id=0  sample_time=0.001000
  EtherCAT PDO Transmit 1 : xpcethercatlib/EtherCAT PDO Transmit   Priority=3  sig_name=RHFE.Outputs.data2  sig_offset=12592  sig_type=uint32  type_size=32  sig_dim=1  device_id=0  sample_time=0.001000
  EtherCAT PDO Transmit 2 : xpcethercatlib/EtherCAT PDO Transmit   Priority=3  sig_name=RHFE.Outputs.data3  sig_offset=12624  sig_type=uint32  type_size=32  sig_dim=1  device_id=0  sample_time=0.001000
  EtherCAT PDO Transmit 3 : xpcethercatlib/EtherCAT PDO Transmit   Priority=3  sig_name=RHFE.Outputs.data4  sig_offset=12656  sig_type=uint32  type_size=32  sig_dim=1  device_id=0  sample_time=0.001000
  EtherCAT PDO Transmit 4 : xpcethercatlib/EtherCAT PDO Transmit   Priority=3  sig_name=RHFE.Outputs.data0  sig_offset=12528  sig_type=uint32  type_size=32  sig_dim=1  device_id=0  sample_time=0.001000
  EtherCAT PDO Transmit 5 : xpcethercatlib/EtherCAT PDO Transmit   Priority=3  sig_name=RHFE.Outputs.data7  sig_offset=12752  sig_type=uint32  type_size=32  sig_dim=1  device_id=0  sample_time=0.001000
  Gain : Gain  Gain=1000  OutDataTypeStr=uint32
  Gain1 : Gain  Gain=1000  OutDataTypeStr=uint32
  Gain2 : Gain  Gain=1000  OutDataTypeStr=uint32
  Kd : Constant  Value=0.1  OutDataTypeStr=double
  Ki : Constant  Value=0  OutDataTypeStr=double
  Kp : Constant  Value=0.11  OutDataTypeStr=double
  Sum : Sum  Inputs=|++
  velocity override : Constant  Value=0  OutDataTypeStr=uint32
  velocity setpoint : Constant  Value=0  OutDataTypeStr=int16
  wires:
  Kd/1 -> Gain2/1
  velocity setpoint/1 -> Data Type Conversion/1
  Kp/1 -> Gain/1
  Constant5/1 -> EtherCAT PDO Transmit 5/1
  Ki/1 -> Gain1/1
  velocity override/1 -> EtherCAT PDO Transmit 3/1
  Constant/1 -> Sum/2
  Data Type Conversion/1 -> Sum/1
  Sum/1 -> Data Type Conversion1/1
  Data Type Conversion1/1 -> EtherCAT PDO Transmit 4/1
  Gain/1 -> "EtherCAT PDO Transmit "/1
  Gain1/1 -> EtherCAT PDO Transmit 1/1
  Gain2/1 -> EtherCAT PDO Transmit 2/1

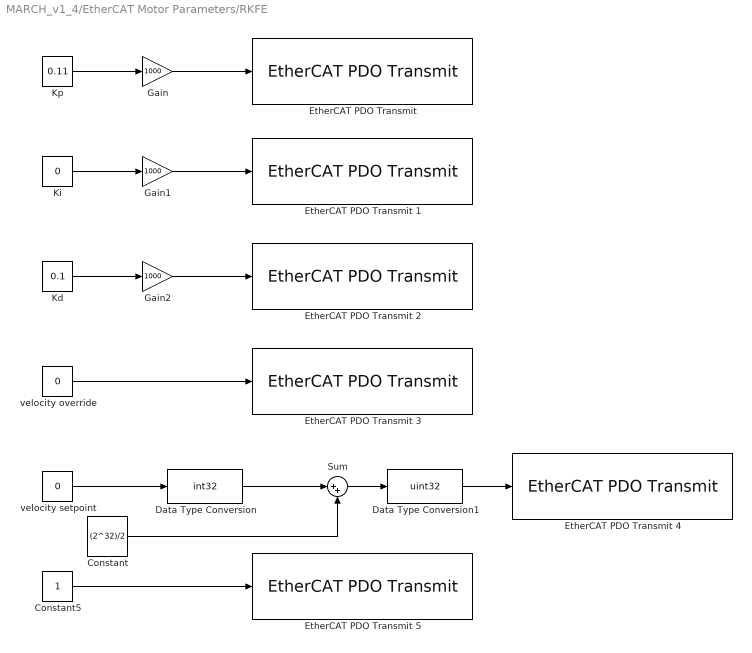
== system MARCH_v1_4/EtherCAT Motor Parameters/RKFE ==
  Constant : Constant  Value=(2^32)/2  VectorParams1D=off  SampleTime=-1
  Constant5 : Constant  OutDataTypeStr=uint32
  Data Type Conversion : DataTypeConversion  OutDataTypeStr=int32
  Data Type Conversion1 : DataTypeConversion  OutDataTypeStr=uint32
  "EtherCAT PDO Transmit " : xpcethercatlib/EtherCAT PDO Transmit   Priority=3  sig_name=RKFE.Outputs.data1  sig_offset=12848  sig_type=uint32  type_size=32  sig_dim=1  device_id=0  sample_time=0.001000
  EtherCAT PDO Transmit 1 : xpcethercatlib/EtherCAT PDO Transmit   Priority=3  sig_name=RKFE.Outputs.data2  sig_offset=12880  sig_type=uint32  type_size=32  sig_dim=1  device_id=0  sample_time=0.001000
  EtherCAT PDO Transmit 2 : xpcethercatlib/EtherCAT PDO Transmit   Priority=3  sig_name=RKFE.Outputs.data3  sig_offset=12912  sig_type=uint32  type_size=32  sig_dim=1  device_id=0  sample_time=0.001000
  EtherCAT PDO Transmit 3 : xpcethercatlib/EtherCAT PDO Transmit   Priority=3  sig_name=RKFE.Outputs.data4  sig_offset=12944  sig_type=uint32  type_size=32  sig_dim=1  device_id=0  sample_time=0.001000
  EtherCAT PDO Transmit 4 : xpcethercatlib/EtherCAT PDO Transmit   Priority=3  sig_name=RKFE.Outputs.data0  sig_offset=12816  sig_type=uint32  type_size=32  sig_dim=1  device_id=0  sample_time=0.001000
  EtherCAT PDO Transmit 5 : xpcethercatlib/EtherCAT PDO Transmit   Priority=3  sig_name=RKFE.Outputs.data7  sig_offset=13040  sig_type=uint32  type_size=32  sig_dim=1  device_id=0  sample_time=0.001000
  Gain : Gain  Gain=1000  OutDataTypeStr=uint32
  Gain1 : Gain  Gain=1000  OutDataTypeStr=uint32
  Gain2 : Gain  Gain=1000  OutDataTypeStr=uint32
  Kd : Constant  Value=0.1  OutDataTypeStr=double
  Ki : Constant  Value=0  OutDataTypeStr=double
  Kp : Constant  Value=0.11  OutDataTypeStr=double
  Sum : Sum  Inputs=|++
  velocity override : Constant  Value=0  OutDataTypeStr=uint32
  velocity setpoint : Constant  Value=0  OutDataTypeStr=int16
  wires:
  Kd/1 -> Gain2/1
  velocity setpoint/1 -> Data Type Conversion/1
  Kp/1 -> Gain/1
  Constant5/1 -> EtherCAT PDO Transmit 5/1
  Ki/1 -> Gain1/1
  velocity override/1 -> EtherCAT PDO Transmit 3/1
  Constant/1 -> Sum/2
  Data Type Conversion/1 -> Sum/1
  Sum/1 -> Data Type Conversion1/1
  Data Type Conversion1/1 -> EtherCAT PDO Transmit 4/1
  Gain/1 -> "EtherCAT PDO Transmit "/1
  Gain1/1 -> EtherCAT PDO Transmit 1/1
  Gain2/1 -> EtherCAT PDO Transmit 2/1

== system MARCH_v1_4/Input Device/EtherCAT Input Device ==
  EtherCAT PDO Receive : xpcethercatlib/EtherCAT PDO Receive  Priority=2  sig_name=LHFE.Inputs.jointAngle  sig_offset=208  sig_type=uint32  type_size=32  sig_dim=1  device_id=0  sample_time=0.001000
  Input Device : Outport
  wires:
  EtherCAT PDO Receive/1 -> Input Device/1

== system MARCH_v1_4/Point&Go/EtherCAT Point&Go ==
  EtherCAT PDO Receive : xpcethercatlib/EtherCAT PDO Receive  Priority=2  sig_name=LHFE.Inputs.jointAngle  sig_offset=208  sig_type=uint32  type_size=32  sig_dim=1  device_id=0  sample_time=0.001000
  Point&Go Data : Outport
  wires:
  EtherCAT PDO Receive/1 -> Point&Go Data/1

== system MARCH_v1_4/Controllers/Continuous Gait/Slider ==

== system MARCH_v1_4/Controllers/Discrete Gait/Slider ==

== system MARCH_v1_4/Controllers/Point & Go/Slider ==

== system MARCH_v1_4/Controllers/Sit and Stand/Slider ==

== system MARCH_v1_4/Controllers/Transition Controller/Slider ==

== system MARCH_v1_4/EtherCAT Joint Setpoints/exoskeleton/EtherCAT Joint Communication ==
  Joint Setpoints : Inport
  Demux : Demux  Outputs=6
  "EtherCAT PDO Transmit " : xpcethercatlib/EtherCAT PDO Transmit   Priority=3  Commented=on  sig_name=LKFE.Outputs.jointSetpoint  sig_offset=496  sig_type=uint32  type_size=32  sig_dim=1  device_id=0  sample_time=0.001000
  EtherCAT PDO Transmit 1 : xpcethercatlib/EtherCAT PDO Transmit   Priority=3  sig_name=RHFE.Outputs.jointSetpoint  sig_offset=12496  sig_type=uint32  type_size=32  sig_dim=1  device_id=0  sample_time=0.001000
  EtherCAT PDO Transmit 2 : xpcethercatlib/EtherCAT PDO Transmit   Priority=3  sig_name=RKFE.Outputs.jointSetpoint  sig_offset=12784  sig_type=uint32  type_size=32  sig_dim=1  device_id=0  sample_time=0.001000
  EtherCAT PDO Transmit 3 : xpcethercatlib/EtherCAT PDO Transmit   Priority=3  Commented=on  sig_name=LHFE.Outputs.data0  sig_offset=240  sig_type=uint32  type_size=32  sig_dim=1  device_id=0  sample_time=0.001000
  EtherCAT PDO Transmit 4 : xpcethercatlib/EtherCAT PDO Transmit   Priority=3  sig_name=LHFE.Outputs.jointSetpoint  sig_offset=208  sig_type=uint32  type_size=32  sig_dim=1  device_id=0  sample_time=0.001000
  EtherCAT PDO Transmit 5 : xpcethercatlib/EtherCAT PDO Transmit   Priority=3  sig_name=LKFE.Outputs.jointSetpoint  sig_offset=496  sig_type=uint32  type_size=32  sig_dim=1  device_id=0  sample_time=0.001000
  wires:
  Demux/5 -> EtherCAT PDO Transmit 4/1
  Demux/6 -> EtherCAT PDO Transmit 5/1
  Demux/4 -> EtherCAT PDO Transmit 3/1
  Demux/1 -> "EtherCAT PDO Transmit "/1
  Demux/2 -> EtherCAT PDO Transmit 1/1
  Joint Setpoints/1 -> Demux/1
  Demux/3 -> EtherCAT PDO Transmit 2/1

== matlab function MARCH_v1_4/Reachability/MATLAB Function ==
  data: q input size=6; q_out output size=6; err output size=6
function [q_out, err] = fcn(q)

joint_limit_min = [-20 -109 -3 -23 -109 -3]'/180*pi;
joint_limit_max = [23 21 121 20 21 121]'/180*pi;

n = size(q,2);
%% Check if all joints are within limits

err = imag(q)~=0 | q<repmat(joint_limit_min,n,1) | q>repmat(joint_limit_max,n,1);
q_out = q;

== matlab function MARCH_v1_4/Controllers/Continuous Gait/Trajectory ==
  data: stepHeight input; q output; stepLength input; q input size=[1 6]; debugOut output; debugIn input
function [q,debugOut]= fcn(stepHeight,stepLength,q,debugIn)
%#codegen

persistent r splineCtrl i trajectory fullStep;

%% Initialize all variables
if(isempty(splineCtrl))
    splineCtrl = splineController();
end


if(isempty(fullStep))
    fullStep = 0;
end

if(isempty(r))
    % Get frequency of the model
    r = robotics();
    r.base = 1;
    
end

if(isempty(i))
    i = 0;
end

if(isempty(trajectory))
    trajectory = [];
end

%% Logic
% Only run this for the beginning of the swing
r.torso_z = debugIn;
if(~i)
    
    % We set the method of whether we want an analytically generated spline
    % or a spline directly from the database.
    % Options: 'analytical' and 'database'
    splineCtrl.setStepLength(stepLength).setStepHeight(stepHeight);
    if(~fullStep)
        trajectory = splineCtrl.method('analytical').getHalfStep();
        fullStep = 1;
    else
        trajectory = splineCtrl.method('analytical').getFullStep();
    end
    
    % Transform the spline to the correct frame based on which foot is
    % swinging
    trajectory = r.transformSpline(trajectory);

    i = i+1;
end

r.point = [trajectory(1,i) trajectory(2,i) trajectory(3,i)];

r.stepPosture();
r.inverseKinematics();

q = r.q;
debugOut = r.torso_z;

% Set final values as initial values for the next iteration
r.refresh();

% Reset iterator after we're done with the trajectory, otherwise we
% increment the counter and continue iterating as simulink continues
% sampling
if( i < (length(trajectory)))
    i = i+1;
else
    i = 0;
    r.switchFoot(r.base);
    r.resetTorso();
end

end

== matlab function MARCH_v1_4/Controllers/Continuous Gait/Torso Trajectory ==
  data: desired input; current input; z output
function z = fcn(desired, current)
%#codegen

persistent trajectory i desiredPersistent;

% Speed at which we home in SAMPLES
samples = 1000;

if (isempty(i))
    i = 0;
    
    % Hack to fix initial condition of delay during init phase
    current = desired;
end

if(isempty(desiredPersistent))
    desiredPersistent = desired;
end

if(isempty(trajectory))
    trajectory = linspace(current,desiredPersistent,samples);
end

if(desiredPersistent ~= desired)
    trajectory = linspace(current,desired,samples);
    desiredPersistent = desired;
    i = 0;
end

if(i < samples)
    i = i+1;
end

z = trajectory(i);

== matlab function MARCH_v1_4/Controllers/Switcher ==
  data: index output; i input; enable output
function [index, enable]= fcn(i)
%#codegen

% This function is supposed to take a state and switch between controllers.
% Currently it directly routes the input argument as the index. In the
% future this can be something different so I have left it open for
% future modifications.

% The u vector represents the controllers. When the vector consists out of
% zeros it will not enable any controller. In the case that an index is set
% to a non zero value, the controller which belongs to that index will be
% enabled.
u = zeros(10,1);

u(i) = 2;

index = i;
enable = u;

== matlab function MARCH_v1_4/EtherCAT Joint Data In/MATLAB Function ==
  data: encoderValue input; angles output; par parameter
function angles = convertToJointAngles(encoderValue, par)
angles = zeros(6,1);

for i = 1:6
    angles(i) = enc2rad(encoderValue(i), i, par);
end

== matlab function MARCH_v1_4/Controllers/Discrete Gait/Torso Trajectory ==
  data: desired input; current input; z output
function z = fcn(desired, current)
%#codegen

persistent trajectory i desiredPersistent;

% Speed at which we home in SAMPLES
samples = 1000;

if (isempty(i))
    i = 0;
    
    % Hack to fix initial condition of delay during init phase
    current = desired;
end

if(isempty(desiredPersistent))
    desiredPersistent = desired;
end

if(isempty(trajectory))
    trajectory = linspace(current,desiredPersistent,samples);
end

if(desiredPersistent ~= desired)
    trajectory = linspace(current,desired,samples);
    desiredPersistent = desired;
    i = 0;
end

if(i < samples)
    i = i+1;
end

z = trajectory(i);

== matlab function MARCH_v1_4/Controllers/Discrete Gait/Trajectory ==
  data: base input; q output; trigger input; q input size=[1 6]; debugOut output; debugIn input
function [q,debugOut]= fcn(base,trigger,q,debugIn)
%#codegen

persistent r splineCtrl i triggerPersistent trajectory fullStep hold;

%% Initialize all variables
if(isempty(splineCtrl))
    splineCtrl = splineController();
end


if(isempty(fullStep))
    fullStep = 0;
end

if(isempty(r))
    % Get frequency of the model
    r = robotics();
    r.base = base;
    
end

if(isempty(hold))
    hold = 0;
end

if(isempty(i))
    i = 0;
end

if(isempty(triggerPersistent))
    triggerPersistent = trigger;
end


if(isempty(trajectory))
    trajectory = [0 0];
end

%% Logic
% Only run this for the beginning of the swing
r.torso_z = debugIn;

% Reset values if trigger is toggled.
if(triggerPersistent ~= trigger)
    r.resetTorso();
    r.base = base;
    i = 0;
    hold = 0;
    triggerPersistent = trigger;
end

if(trigger == -1)
   fullStep = 0; 
end

% Hold exoskeleton in same position after a single step
if(hold)
    debugOut = r.torso_z;
    q = r.q;
    return
end

if(~i)
    
    % We set the method of whether we want an analytically generated spline
    % or a spline directly from the database.
    % Options: 'analytical' and 'database'
    if(~fullStep)
        trajectory = splineCtrl.method('analytical').getHalfStep();
        fullStep = 1;
    else
        trajectory = splineCtrl.method('analytical').getFullStep();
    end
    
    % Transform the spline to the correct frame based on which foot is
    % swinging
    trajectory = r.transformSpline(trajectory);
    
    i = i+1;
end

r.point = [trajectory(1,i) trajectory(2,i) trajectory(3,i)];

r.stepPosture();
r.inverseKinematics();

q = r.q;
debugOut = r.torso_z;

% Set final values as initial values for the next iteration
r.refresh();

% Reset iterator after we're done with the trajectory, otherwise we
% increment the counter and continue iterating as simulink continues
% sampling
if( i < (length(trajectory)))
    i = i+1;
else
    hold = 1;
end

end

== matlab function MARCH_v1_4/Controllers/Transition Controller/Torso Trajectory ==
  data: desired input; current input; z output
function z = fcn(desired, current)
%#codegen

persistent trajectory i desiredPersistent;

% Speed at which we home in SAMPLES
samples = 1000;

if (isempty(i))
    i = 0;
    
    % Hack to fix initial condition of delay during init phase
    current = desired;
end

if(isempty(desiredPersistent))
    desiredPersistent = desired;
end

if(isempty(trajectory))
    trajectory = linspace(current,desiredPersistent,samples);
end

if(desiredPersistent ~= desired)
    trajectory = linspace(current,desired,samples);
    desiredPersistent = desired;
    i = 0;
end

if(i < samples)
    i = i+1;
end

z = trajectory(i);
